simulink model "no"  (R2016a)
settings: Solver=VariableStepAuto  StartTime=0.0  StopTime=inf  FixedStep=0.005  RelTol=1e-3
PreLoadFcn:
  | load('param.mat')
libraries: LibrarySimulinkSAS x3, realtime_pacer_lib x1
settings Model: Creator=M  LastModifiedBy=M

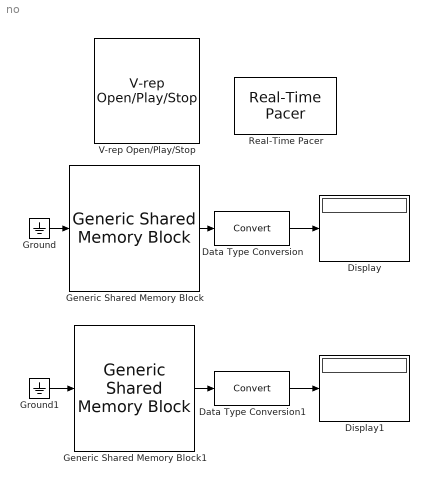
== system no ==
  Data Type Conversion : DataTypeConversion
  Data Type Conversion1 : DataTypeConversion
  Display : Display
  Display1 : Display
  Generic Shared Memory Block : LibrarySimulinkSAS/Generic Shared Memory Block  nombre='vel_torq_left'  dispositivo=1  vecE=[1]  vecS=[2]  tipoE=['f']  tipoS=['f']  ts=-1
  Generic Shared Memory Block1 : LibrarySimulinkSAS/Generic Shared Memory Block  nombre='vel_torq_right'  dispositivo=2  vecE=[1]  vecS=[2]  tipoE=['f']  tipoS=['f']  ts=-1
  Ground : Ground
  Ground1 : Ground
  Real-Time Pacer : realtime_pacer_lib/Real-Time Pacer  simTimePerRealTime=1
  V-rep Open/Play/Stop : LibrarySimulinkSAS/V-rep Open//Play//Stop  scene='cuboidVrep.ttt'
  wires:
  Ground/1 -> Generic Shared Memory Block/1
  Generic Shared Memory Block1/1 -> Data Type Conversion1/1
  Ground1/1 -> Generic Shared Memory Block1/1
  Generic Shared Memory Block/1 -> Data Type Conversion/1
  Data Type Conversion/1 -> Display/1
  Data Type Conversion1/1 -> Display1/1
